simulink model "RegularCheckoutsOnly"  (R2020a)
settings: Solver=VariableStepAuto  StartTime=0.0  StopTime=500000  RelTol=1e-3
InitFcn:
  | SimulationParameters
values from neighbouring files (symbols this model uses):
  NumRegularCheckouts = 15    [SimulationParameters.m]
  RegularQueueCapacity = 7    [SimulationParameters.m]
undefined symbols (not defined in the file or in its folder): m, n
libraries: dspindex x1, dspstat3 x1
settings Model: Creator=jggam  LastModifiedBy=jggam

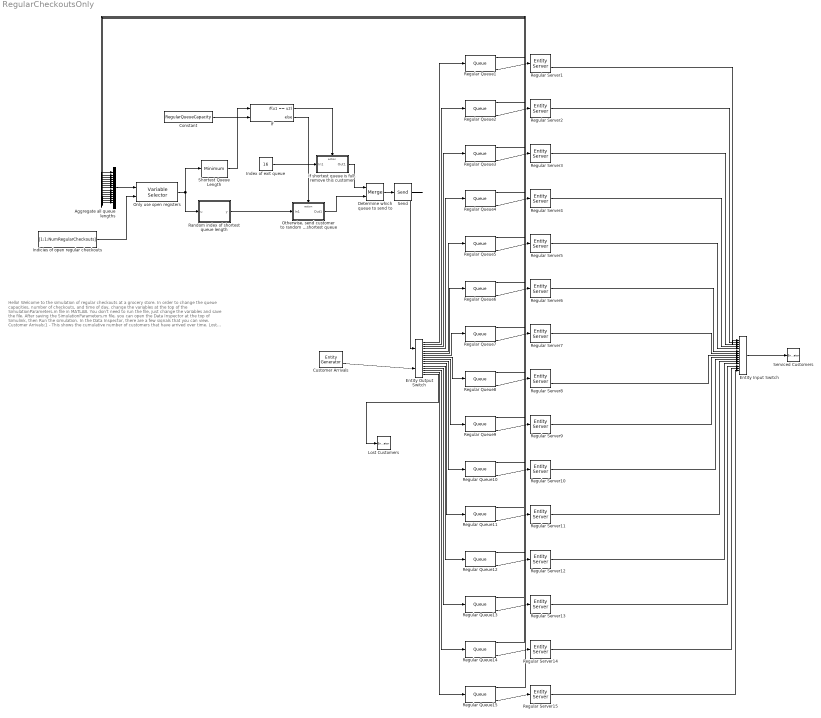
== system RegularCheckoutsOnly ==
  note: Hello! Welcome to the simulation of regular checkouts at a grocery store.
      | In order to change the queue capacities, number of checkouts, and time of day,
      | 	change the variables at the top of the SimulationParameters.m file in MATLAB.
      | You don't need to run the file, just change the variables and save the file.
      | After saving the SimulationParameters.m file, you can open the Data Inspector at the top of Simulink,
      | 	then Run the simulation.
      |
      | In the Data Inspector, there are a few signals that you can view.
      | 	Customer Arrivals:1 - This shows the cumulative number of customers that have arrived over time.
      | 	Lost Customers:1 - This shows the cumulative number of customers that have left the store because the queues were all full over time.
      | 	Serviced Customers:1 - This shows the cumulative number of customers that have been serviced over time (throughput).
      | 	Regular Queue 1: Current # of customers
      | 	Regular Queue 1: Average wait time
      | 	Regular Queue 1: Average # of customers
      | 	Regular Queue 2: Current # of customers
      | 	Regular Queue 2: Average wait time
      | 	Regular Queue 2: Average # of customers
      | 	Regular Queue 3: Current # of customers
      | 	Regular Queue 3: Average wait time
      | 	Regular Queue 3: Average # of customers
  Aggregate all queue lengths : Concatenate  NumInputs=15
  Constant : Constant  Value=RegularQueueCapacity
  Customer Arrivals : EntityGenerator  OutputPortMessageModes=n,m  TimeSource=MATLAB action  Period=0.5  IntergenerationTimeAction=dt = arrivalTime(RandArrivalTimesDist);  GenerateEntityAtSimulationStart=off  GenerateAction=|  AttributeName=NumberOfItems|RandomChoice  AttributeInitialValue=1|1  NumberEntitiesDeparted=on  EntityType=Structured  EntityTypeName=Entity
      | entity.NumberOfItems = numberOfItems(RandItemsDist);
      | if rand() < 0.3 && entity.NumberOfItems <= 5
      |     entity.RandomChoice = 2;
      | else
      |     entity.RandomChoice = 1;
      | end
      settings: OutputPortMap=o0,o3
  Determine which queue to send to : Merge
  Entity Input Switch : EntityInputSwitch  InputPortMessageModes=m,m,m,m,m,m,m,m,m,m,m,m,m,m,m  OutputPortMessageModes=m  NumberInputPorts=15
      settings: InputPortMap=u1,u2,u3,u4,u5,u6,u7,u8,u9,u10,u11,u12,u13,u14,u15
  Entity Output Switch : EntityOutputSwitch  InputPortMessageModes=m,m  OutputPortMessageModes=m,m,m,m,m,m,m,m,m,m,m,m,m,m,m,m  NumberOutputPorts=16  SwitchingCriterion=From control port  SwitchAttributeName=Attribute1  InitialPortSelection=randi(NumRegularCheckouts)
      settings: InputPortMap=u0,u1  OutputPortMap=o0,o1,o2,o3,o4,o5,o6,o7,o8,o9,o10,o11,o12,o13,o14,o15
  If : If  NumInputs=2  IfExpression=u1 == u2  ZeroCross=off
  "If shortest queue is full, remove this customer" : Subsystem  TreatAsAtomicUnit=on
  Index of exit queue : Constant  Value=16
  Indicies of open regular checkouts : Constant  Value=[1:1:NumRegularCheckouts]
  Lost Customers : EntityTerminator  InputPortMessageModes=m  NumberEntitiesArrived=on
      settings: OutputPortMap=o0
  Only use open registers : dspindex/Variable Selector  NumInputs=1  rowsOrCols=Rows  IdxMode=Variable  Elements=[1 3]  ZerOneIdxMode=One-based  errmode=Clip Index  FillMode=on  FillValues=0
  "Otherwise, send customer to random shortest queue" : Subsystem  TreatAsAtomicUnit=on
  Random index of shortest queue length : MATLAB Function  TreatAsAtomicUnit=on
  Regular Queue{1..15} (15 alike) : Queue  InputPortMessageModes=m  OutputPortMessageModes=n,n,n,m  Capacity=RegularQueueCapacity  NumberEntitiesInBlock=on  AverageWait=on  AverageQueueLength=on
      settings: OutputPortMap=o1,o2,o3,o5
  Regular Server1 : EntityServer  InputPortMessageModes=m  OutputPortMessageModes=n,m  Capacity=1  ServiceTimeSource=MATLAB action  ServiceTimeValue=1.75  ServiceTimeAction=dt = regularServiceTime(RandRegularServiceTimesDist);  AverageWait=on
      settings: OutputPortMap=o4,o9
  Regular Server{2..7,9..15} (13 alike) : EntityServer  InputPortMessageModes=m  OutputPortMessageModes=m  Capacity=1  ServiceTimeSource=MATLAB action  ServiceTimeValue=1.75  ServiceTimeAction=dt = regularServiceTime(RandRegularServiceTimesDist);
  Regular Server8 : EntityServer  InputPortMessageModes=m  OutputPortMessageModes=n,m  Capacity=1  ServiceTimeSource=MATLAB action  ServiceTimeValue=1.75  ServiceTimeAction=dt = regularServiceTime(RandRegularServiceTimesDist);  AverageWait=on
      settings: OutputPortMap=o4,o9
  Send : Send  OutputPortMessageModes=m
  Serviced Customers : EntityTerminator  InputPortMessageModes=m  NumberEntitiesArrived=on
      settings: OutputPortMap=o0
  Shortest Queue Length : dspstat3/Minimum  operation=minimum  fcn=Value  indexBase=One  operateOver=Entire input  Dimension=1  InputProcessing=Columns as channels (frame based)  reset=None  roiEnable=off  roiType=Rectangles  roiPortion=Entire ROI  roiOutput=Individual statistics for each ROI  roiFlag=off  roundingMode=Floor  overflowMode=off
      settings: SourceProductBaseCode=DS
  wires:
  Regular Queue1/4 -> Regular Server1/1
  Entity Input Switch/1 -> Serviced Customers/1
  Send/1 -> Entity Output Switch/1
  Customer Arrivals/2 -> Entity Output Switch/2
  Regular Queue1/1 -> Aggregate all queue lengths/1
  Regular Queue2/4 -> Regular Server2/1
  Regular Queue3/4 -> Regular Server3/1
  Regular Queue4/4 -> Regular Server4/1
  Regular Queue5/4 -> Regular Server5/1
  Regular Queue6/4 -> Regular Server6/1
  Regular Queue7/4 -> Regular Server7/1
  Regular Queue8/4 -> Regular Server8/1
  Regular Queue9/4 -> Regular Server9/1
  Regular Queue10/4 -> Regular Server10/1
  Regular Queue11/4 -> Regular Server11/1
  Regular Queue12/4 -> Regular Server12/1
  Regular Queue13/4 -> Regular Server13/1
  Regular Queue14/4 -> Regular Server14/1
  Regular Queue15/4 -> Regular Server15/1
  Regular Server2/1 -> Entity Input Switch/2
  Regular Server3/1 -> Entity Input Switch/3
  Regular Server4/1 -> Entity Input Switch/4
  Regular Server5/1 -> Entity Input Switch/5
  Regular Server6/1 -> Entity Input Switch/6
  Regular Server7/1 -> Entity Input Switch/7
  Regular Server8/2 -> Entity Input Switch/8
  Regular Server9/1 -> Entity Input Switch/9
  Regular Server10/1 -> Entity Input Switch/10
  Regular Server11/1 -> Entity Input Switch/11
  Regular Server12/1 -> Entity Input Switch/12
  Regular Server13/1 -> Entity Input Switch/13
  Regular Server14/1 -> Entity Input Switch/14
  Regular Server15/1 -> Entity Input Switch/15
  Regular Queue2/1 -> Aggregate all queue lengths/2
  Regular Queue3/1 -> Aggregate all queue lengths/3
  Regular Queue4/1 -> Aggregate all queue lengths/4
  Regular Queue5/1 -> Aggregate all queue lengths/5
  Regular Queue6/1 -> Aggregate all queue lengths/6
  Regular Queue7/1 -> Aggregate all queue lengths/7
  Regular Queue8/1 -> Aggregate all queue lengths/8
  Regular Queue9/1 -> Aggregate all queue lengths/9
  Entity Output Switch/1 -> Regular Queue1/1
  Entity Output Switch/2 -> Regular Queue2/1
  Entity Output Switch/3 -> Regular Queue3/1
  Entity Output Switch/4 -> Regular Queue4/1
  Entity Output Switch/5 -> Regular Queue5/1
  Entity Output Switch/6 -> Regular Queue6/1
  Entity Output Switch/7 -> Regular Queue7/1
  Entity Output Switch/8 -> Regular Queue8/1
  Entity Output Switch/9 -> Regular Queue9/1
  Entity Output Switch/10 -> Regular Queue10/1
  Entity Output Switch/11 -> Regular Queue11/1
  Entity Output Switch/12 -> Regular Queue12/1
  Entity Output Switch/13 -> Regular Queue13/1
  Entity Output Switch/14 -> Regular Queue14/1
  Entity Output Switch/15 -> Regular Queue15/1
  Entity Output Switch/16 -> Lost Customers/1
  Shortest Queue Length/1 -> If/1
  If/1 -> "If shortest queue is full, remove this customer"/Action
  If/2 -> "Otherwise, send customer to random shortest queue"/Action
  Regular Server1/2 -> Entity Input Switch/1
  Determine which queue to send to/1 -> Send/1
  Index of exit queue/1 -> "If shortest queue is full, remove this customer"/1(In1)
  "If shortest queue is full, remove this customer"/1(Out1) -> Determine which queue to send to/1
  Random index of shortest queue length/1(y) -> "Otherwise, send customer to random shortest queue"/1(In1)
  Regular Queue10/1 -> Aggregate all queue lengths/10
  Regular Queue11/1 -> Aggregate all queue lengths/11
  Regular Queue12/1 -> Aggregate all queue lengths/12
  Regular Queue13/1 -> Aggregate all queue lengths/13
  Regular Queue14/1 -> Aggregate all queue lengths/14
  Regular Queue15/1 -> Aggregate all queue lengths/15
  "Otherwise, send customer to random shortest queue"/1(Out1) -> Determine which queue to send to/2
  Constant/1 -> If/2
  Aggregate all queue lengths/1 -> Only use open registers/1
  Only use open registers/1 -> Random index of shortest queue length/1(u), Shortest Queue Length/1
  Indicies of open regular checkouts/1 -> Only use open registers/2

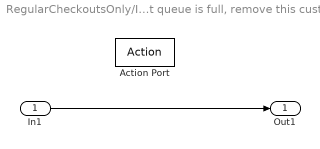
== system RegularCheckoutsOnly/If shortest queue is full, remove this customer ==
  In1 : Inport
  Action Port : ActionPort  ActionPortLabel=if(u1 == u2)
  Out1 : Outport
  wires:
  In1/1 -> Out1/1

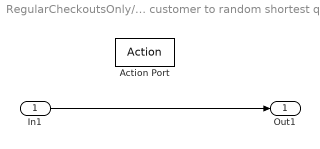
== system RegularCheckoutsOnly/Otherwise, send customer to random shortest queue ==
  In1 : Inport
  Action Port : ActionPort  ActionPortLabel=else
  Out1 : Outport
  wires:
  In1/1 -> Out1/1

== matlab function RegularCheckoutsOnly/Random index of shortest queue length ==
  data: u input; y output
function y = findAllMinLengthIndices(u)

indicies = find(u == min(u));
y = indicies(randi(length(indicies)));
